simulink subsystem "EV1_ThorneFleissner"  (R2020b)
settings: Solver=VariableStepAuto  StartTime=0.0  StopTime=10.0  RelTol=1e-3
settings Model: Creator=rthom  LastModifiedBy=rthom

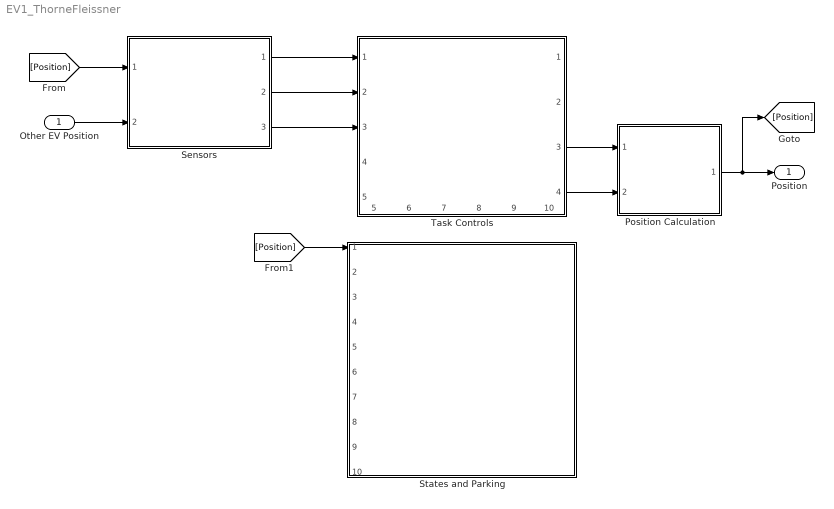
== system EV1_ThorneFleissner ==
  Other EV Position : Inport
  Position Calculation : Subsystem  ReferencedSubsystem=Position_Calculation_ThorneFleissner
  Sensors : Subsystem  ReferencedSubsystem=Sensors_ThorneFleissner
  States and Parking : Subsystem  ReferencedSubsystem=Parking_ThorneFleissner
  Task Controls : Subsystem  ReferencedSubsystem=Task_Controls_ThorneFleissner
      settings: PortSchema="{\"entries\":[{\"content\":{\"sides\":[{\"content\":{\"connectorIds\":[\"In1\",\"In2\",\"In3\",\"In4\",\"In5\"]},\"type\":\"ConnectorPlacement.EquallySpacedRectSide\",\"uuid\":\"3c64813c-625d-49d1-ae67-306451c3c1fa\"},{\"content\":{\"connectorIds\":[\"Out1\",\"Out2\",\"Out3\",\"Out4\"],\"side\":\"RIGHT\"},\"type\":\"ConnectorPlacement.EquallySpacedRectSide\",\"uuid\":\"91793cf5-b7a0-4d71-a2c0-83cdd43afca2\"},{\"content\":{\"connectorIds\":[],\"side\":\"TOP\"},\"type\":\"ConnectorPlacement.EquallySpacedRectSide\",\"uuid\":\"5300aefe-28d7-4142-9759-b53f625cf082\"},{\"content\":{\"connectorIds\":[\"Out5\",\"Out6\",\"Out7\",\"Out8\",\"Out9\",\"Out10\"],\"side\":\"BOTTOM\"},\"type\":\"ConnectorPlacement.EquallySpacedRectSide\",\"uuid\":\"7541b0a2-c079-4b1b-9276-8e4ee5949dfd\"},{\"content\":{\"connectorIds\":[],\"side\":\"HIDDEN\"},\"type\":\"ConnectorPlacement.EquallySpacedRectSide\",\"uuid\":\"d0ef4c96-52b1-4a81-ac1e-c57b650a37a1\"}]},\"type\":\"ConnectorPlacement.EquallySpacedConnector\",\"uuid\":\"d02aae7f-e4d5-4935-81ce-eef5c5855771\"}],\"packageUris\":[\"http://schema.mathworks.com/mf0/Connector/R2020b\"],\"version\":\"1.0\"}"
  Position : Outport
  wires:
  Position Calculation/1 -> Position/1, [Position]
  Task Controls/3 -> Position Calculation/1
  Task Controls/4 -> Position Calculation/2
  Sensors/3 -> Task Controls/3
  Sensors/1 -> Task Controls/1
  Sensors/2 -> Task Controls/2
  Other EV Position/1 -> Sensors/2
  [Position] -> Sensors/1
  [Position] -> States and Parking/1
